simulink model "manual_steer"  (R2022b)
settings: Solver=ode4  StartTime=0.0  StopTime=100  RelTol=1e-3
model workspace (MAT data in the model file):
  x2xx = 0
undefined symbols (not defined in the file or in its folder): axle_rate_limit, BRAKE, brake_lag, brake_rate, DRIVE, KDspd, KIspd, KPspd, Lspd, Nspd, PARSa, PARSu, Q0, QD0, RW, Tb, Tmc, TOTALMASS, Tst, Uspd, v_ref
libraries: CarMaker4SL x72, slpidlib x4, TruckMaker4SL x1, simulink x1
(part 5 of 5)

== matlab function manual_steer/double sat_tyre general model/double-general-nonlineartyre-nonlinear-variable-matrix/M ==
  data: M output; q input
function M = calculate_M(q)

psi1 = q(3);
psi2 = q(4);
psi3 = q(5);

m1 = 11142;
m3 = 11142;
m2 = 7651; 
l_j1j2 = 11.4;
l_j2j3 = 9.4;
l_j1g1 = 5.862; 
l_j2g2 = 4.643; 
l_j3g3 = 5.538; 
iz1 = 143570; 
iz3 = 143570; 
iz2 = 37800;

l_kj = [l_j1g1, l_j1j2, l_j1j2;
             0, l_j2g2, l_j2j3;
             0,      0, l_j3g3;];
delta_kj = eye(3);
Jc = zeros(3, 5, 3);
for j = 1:3
    Jc(:, :, j) = [1, 0,  l_kj(1, j) * sin(psi1),  l_kj(2, j) * sin(psi2),  l_kj(3, j) * sin(psi3);
          0, 1, -l_kj(1, j) * cos(psi1), -l_kj(2, j) * cos(psi2), -l_kj(3, j) * cos(psi3);
          0, 0,          delta_kj(1, j),          delta_kj(2, j),          delta_kj(3, j);];
end

mj = [m1, m2, m3]';
izj = [iz1, iz2, iz3]';
Mj = zeros(3, 3, 3);
for j = 1:3
    Mj(:, :, j) = diag([mj(j), mj(j), izj(j)]);
end

M = zeros(5, 5);
for j = 1:3
    M = M + Jc(:, :, j)' * Mj(:, :, j) * Jc(:, :, j);
end

end

== matlab function manual_steer/double sat_tyre general model/double-general-nonlineartyre-nonlinear-variable-matrix/Tau_tire ==
  data: q input; qd input; delta input; Fx input; Tau_tire output; Alpha output
function [Tau_tire, Alpha] = calculate_Tau_tire(q, qd, delta, Fx)

% coefficient

l_j1j2 = 11.4;
l_j2j3 = 9.4;
l_j1a1 = 2.5;
l_j1a2 = 4;
l_j1a3 = 9.9;
l_j2a4 = 1.5;
l_j2a5 = 7.9;
l_j3a6 = 1.5;
l_j3a7 = 7.4;
l_j3a8 = 8.9;
h11 = 0.9625;
h12 = 0.9625;
h13 = 0.98;
h21 = 0.98; 
h22 = 0.98;
h31 = 0.98;
h32 = 0.9625;
h33 = 0.9625;

x = q(1);
y = q(2);
psi1 = q(3);
psi2 = q(4);
psi3 = q(5);
xd = qd(1);
yd = qd(2);
psi1d = qd(3);
psi2d = qd(4);
psi3d = qd(5);

psij = [psi1, psi2, psi3]';
Rot_w2v = zeros(2, 2, 3);
for i = 1:3
    Rot_w2v(:, :, i) = [cos(psij(i)), -sin(psij(i));
                        sin(psij(i)), cos(psij(i));];
end

Rot_v2t = zeros(2, 2, 8);
for i = 1:8
    Rot_v2t(:, :, i) = [cos(delta(i)), -sin(delta(i));
                        sin(delta(i)), cos(delta(i));];
end

xj = zeros(3, 1);
yj = zeros(3, 1);
xj(1) = x;
yj(1) = y;
xj(2) = x - l_j1j2*cos(psi1);
yj(2) = y - l_j1j2*sin(psi1);
xj(3) = x - l_j1j2*cos(psi1) - l_j2j3*cos(psi2);
yj(3) = y - l_j1j2*sin(psi1) - l_j2j3*sin(psi2);

u = zeros(2, 3);
n = zeros(2, 3);
for i = 1:3
    u(:, i)=[cos(q(i + 2)), sin(q(i + 2))]';
    n(:, i)=[-sin(q(i + 2)), cos(q(i + 2))]';
end

IU = [1, 1, 1, 2, 2, 3, 3, 3]';
l_ja = [l_j1a1, l_j1a2, l_j1a3, l_j2a4, l_j2a5, l_j3a6, l_j3a7, l_j3a8]';
ha = [h11, h12, h13, h21, h22, h31, h32, h33]';

L_long1 = [cos(psi1), cos(psi1), cos(psi1), cos(psi2), cos(psi2), cos(psi3), cos(psi3), cos(psi3);
           sin(psi1), sin(psi1), sin(psi1), sin(psi2), sin(psi2), sin(psi3), sin(psi3), sin(psi3);
           -h11, -h12, -h13, l_j1j2*sin(psi1-psi2), l_j1j2*sin(psi1-psi2), l_j1j2*sin(psi1-psi3), l_j1j2*sin(psi1-psi3), l_j1j2*sin(psi1-psi3);
           0, 0, 0, -h21, -h22, l_j2j3*sin(psi2-psi3), l_j2j3*sin(psi2-psi3), l_j2j3*sin(psi2-psi3);
           0, 0, 0, 0, 0, -h31, -h32, -h33;];

L_long2 = [cos(psi1), cos(psi1), cos(psi1), cos(psi2), cos(psi2), cos(psi3), cos(psi3), cos(psi3);
           sin(psi1), sin(psi1), sin(psi1), sin(psi2), sin(psi2), sin(psi3), sin(psi3), sin(psi3);
           h11, h12, h13, l_j1j2*sin(psi1-psi2), l_j1j2*sin(psi1-psi2), l_j1j2*sin(psi1-psi3), l_j1j2*sin(psi1-psi3), l_j1j2*sin(psi1-psi3);
           0, 0, 0, h21, h22, l_j2j3*sin(psi2-psi3), l_j2j3*sin(psi2-psi3), l_j2j3*sin(psi2-psi3);
           0, 0, 0, 0, 0, h31, h32, h33;];

L_lat1 = [-sin(psi1), -sin(psi1), -sin(psi1), -sin(psi2), -sin(psi2), -sin(psi3), -sin(psi3), -sin(psi3);
          cos(psi1), cos(psi1), cos(psi1), cos(psi2), cos(psi2), cos(psi3), cos(psi3), cos(psi3);
          -l_j1a1, -l_j1a2, -l_j1a3, -l_j1j2*cos(psi1-psi2), -l_j1j2*cos(psi1-psi2), -l_j1j2*cos(psi1-psi3), -l_j1j2*cos(psi1-psi3), -l_j1j2*cos(psi1-psi3);
          0, 0, 0, -l_j2a4, -l_j2a5, -l_j2j3*cos(psi2-psi3), -l_j2j3*cos(psi2-psi3), -l_j2j3*cos(psi2-psi3);
          0, 0, 0, 0, 0, -l_j3a6, -l_j3a7, -l_j3a8;];

L_lat2 = [-sin(psi1), -sin(psi1), -sin(psi1), -sin(psi2), -sin(psi2), -sin(psi3), -sin(psi3), -sin(psi3);
          cos(psi1), cos(psi1), cos(psi1), cos(psi2), cos(psi2), cos(psi3), cos(psi3), cos(psi3);
          -l_j1a1, -l_j1a2, -l_j1a3, -l_j1j2*cos(psi1-psi2), -l_j1j2*cos(psi1-psi2), -l_j1j2*cos(psi1-psi3), -l_j1j2*cos(psi1-psi3), -l_j1j2*cos(psi1-psi3);
          0, 0, 0, -l_j2a4, -l_j2a5, -l_j2j3*cos(psi2-psi3), -l_j2j3*cos(psi2-psi3), -l_j2j3*cos(psi2-psi3);
          0, 0, 0, 0, 0, -l_j3a6, -l_j3a7, -l_j3a8;];

Delta_c = zeros(8, 8);
Delta_s = zeros(8, 8);
for i = 1:8
    Delta_c(i, i) = cos(delta(i));
    Delta_s(i, i) = sin(delta(i));
end

vxj = zeros(3, 1);
vyj = zeros(3, 1);
vxj(1) = xd;
vyj(1) = yd;
vxj(2) = xd + l_j1j2*sin(psi1)*psi1d;
vyj(2) = yd - l_j1j2*cos(psi1)*psi1d;
vxj(3) = xd + l_j1j2*sin(psi1)*psi1d + l_j2j3*sin(psi2)*psi2d;
vyj(3) = yd - l_j1j2*cos(psi1)*psi1d - l_j2j3*cos(psi2)*psi2d;
va1 = zeros(2, 8);
va2 = zeros(2, 8);
psidj = [psi1d, psi2d, psi3d]';
for i = 1:8
    va1(:, i) = [vxj(IU(i)); vyj(IU(i))] - n(:, IU(i))*l_ja(i)*psidj(IU(i)) + (-1)*u(:, IU(i))*ha(i)*psidj(IU(i));
    va2(:, i) = [vxj(IU(i)); vyj(IU(i))] - n(:, IU(i))*l_ja(i)*psidj(IU(i)) + u(:, IU(i))*ha(i)*psidj(IU(i));
end

va1_v = zeros(2, 8);
va2_v = zeros(2, 8);
for i = 1:8
    va1_v(:, i) = inv(Rot_w2v(:, :, IU(i)))*va1(:, i);
    va2_v(:, i) = inv(Rot_w2v(:, :, IU(i)))*va2(:, i);
end

beta1 = zeros(8, 1);
beta2 = zeros(8, 1);
for i = 1:8
    beta1(i) = atan2(va1_v(2, i), va1_v(1, i));
    beta2(i) = atan2(va2_v(2, i), va2_v(1, i));
end

% magic formula
% 魔术公式参数
A = [1.65, -34, 1250, 4535, 12.8, 0.00501, -0.02103,  0.77394, ...
     0.0022890, 0.013442, 0.003709, 19.1656, 1.21356, 6.26206]';

% 轮胎垂向载荷 kN
Fz = 30000 / 1000;

Fy1 = zeros(8, 1);
Fy2 = zeros(8, 1);
gamma = 0;
for i = 1:8
    alpha = (delta(i) - beta1(i)) * 180 / pi;
    Sh = A(10) * Fz + A(11) + A(9) * gamma;
    Sv = A(12) * Fz * gamma + A(13) * Fz + A(14);
    C = A(1);
    D = A(2) * Fz ^ 2 + A(3) * Fz;
    BCD = A(4) * sin(2 * atan(Fz / A(5))) * (1 - A(6) * abs(gamma));
    B = BCD / (C * D);
    E = A(7) * Fz + A(8);
    x = alpha; % + Sh;
    % 轮胎侧向力
    Fy1(i) = D * sin(C * atan(B * x - E * (B * x - atan(B * x)))); % + Sv;
end
for i = 1:8
    alpha = (delta(i) - beta2(i)) * 180 / pi;
    Sh = A(10) * Fz + A(11) + A(9) * gamma;
    Sv = A(12) * Fz * gamma + A(13) * Fz + A(14);
    C = A(1);
    D = A(2) * Fz ^ 2 + A(3) * Fz;
    BCD = A(4) * sin(2 * atan(Fz / A(5))) * (1 - A(6) * abs(gamma));
    B = BCD / (C * D);
    E = A(7) * Fz + A(8);
    x = alpha; % + Sh;
    % 轮胎侧向力
    Fy2(i) = D * sin(C * atan(B * x - E * (B * x - atan(B * x)))); % + Sv;
end

Tau_tire = L_long1 * (Delta_c * Fx / 2 - Delta_s * Fy1) ...
         + L_long2 * (Delta_c * Fx / 2 - Delta_s * Fy2) ...
         + L_lat1 * (Delta_s * Fx / 2 + Delta_c * Fy1) ...
         + L_lat2 * (Delta_s * Fx / 2 + Delta_c * Fy2);

beta = (beta1 + beta2) / 2;
Alpha = delta - beta;

end

== matlab function manual_steer/double sat_tyre general model/double-general-nonlineartyre-nonlinear-variable-matrix/qdd ==
  data: M input; C input; D input; qd input; Q input; qdd output
function qdd = calculate_qdd(M, C, D, qd, Q)

qdd = inv(M)*(Q - C * qd - D * qd);

end

== matlab function manual_steer/single sat_tyre general model/single-general-lineartyre-variable/D ==
  data: D output
function D = calculate_D()

d1 = 10000;
d2 = 10000;

delta_kj = eye(3);
dj = [0, d1, d2, 0]';
D = zeros(5);

for k = 1:5
    for l = 1:5
        if k > 2 && l > 2
            if  l == k
                D(k, l) = (1 - delta_kj(1, k-2))*dj(k - 2) + (1 - delta_kj(3, k-2))*dj(k - 1);
            elseif l == k-1
                D(k, l) = -(1 - delta_kj(1, k-2))*dj(k - 2);
            elseif l == k+1
                D(k, l) = -(1 - delta_kj(3, k-2))*dj(k - 1);
            else
                D(k, l) = 0;
            end
        end
    end
end

end

== matlab function manual_steer/single sat_tyre general model/single-general-lineartyre-variable/M ==
  data: M output; q input
function M = calculate_M(q)

psi1 = q(3);
psi2 = q(4);
psi3 = q(5);

m1 = 11142;
m3 = 11142;
m2 = 7651; 
l_j1j2 = 11.4;
l_j2j3 = 9.4;
l_j1g1 = 5.862; 
l_j2g2 = 4.643; 
l_j3g3 = 5.538; 
iz1 = 143570; 
iz3 = 143570; 
iz2 = 37800;

l_kj = [l_j1g1, l_j1j2, l_j1j2;
             0, l_j2g2, l_j2j3;
             0,      0, l_j3g3;];
delta_kj = eye(3);
Jc = zeros(3, 5, 3);
for j = 1:3
    Jc(:, :, j) = [1, 0,  l_kj(1, j) * sin(psi1),  l_kj(2, j) * sin(psi2),  l_kj(3, j) * sin(psi3);
          0, 1, -l_kj(1, j) * cos(psi1), -l_kj(2, j) * cos(psi2), -l_kj(3, j) * cos(psi3);
          0, 0,          delta_kj(1, j),          delta_kj(2, j),          delta_kj(3, j);];
end

mj = [m1, m2, m3]';
izj = [iz1, iz2, iz3]';
Mj = zeros(3, 3, 3);
for j = 1:3
    Mj(:, :, j) = diag([mj(j), mj(j), izj(j)]);
end

M = zeros(5, 5);
for j = 1:3
    M = M + Jc(:, :, j)' * Mj(:, :, j) * Jc(:, :, j);
end

end

== matlab function manual_steer/double sat_tyre general model/ Motion Controller1/discrete-time subsystem/MATLAB Function ==
  data: str1 input; y output; PARSa input
function y = StrMux(str1,PARSa)
%distribute steering from driver (and auto steer in future versions)
y=PARSa(:,6);
y=y*str1;
end

== matlab function manual_steer/single sat_tyre general model/single-general-lineartyre-variable/Tau_tire ==
  data: q input; qd input; delta input; Fx input; Tau_tire output; Alpha output
function [Tau_tire, Alpha] = calculate_Tau_tire(q, qd, delta, Fx)

% coefficient

l_j1j2 = 11.4;
l_j2j3 = 9.4;
l_j1a1 = 2.5;
l_j1a2 = 4;
l_j1a3 = 9.9;
l_j2a4 = 1.5;
l_j2a5 = 7.9;
l_j3a6 = 1.5;
l_j3a7 = 7.4;
l_j3a8 = 8.9;
h11 = 0;
h12 = 0;
h13 = 0;
h21 = 0; 
h22 = 0;
h31 = 0;
h32 = 0;
h33 = 0;

ca_T = 3065;
ca1 = ca_T;
ca2 = ca_T;
ca3 = ca_T;
ca4 = ca_T;
ca5 = ca_T;
ca6 = ca_T;
ca7 = ca_T;
ca8 = ca_T;

psi1 = q(3);
psi2 = q(4);
psi3 = q(5);
xd = qd(1);
yd = qd(2);
psi1d = qd(3);
psi2d = qd(4);
psi3d = qd(5);

psij = [psi1, psi2, psi3]';
Rot_w2v = zeros(2, 2, 3);
for i = 1:3
    Rot_w2v(:, :, i) = [cos(psij(i)), -sin(psij(i));
                        sin(psij(i)), cos(psij(i));];
end

Rot_v2t = zeros(2, 2, 8);
for i = 1:8
    Rot_v2t(:, :, i) = [cos(delta(i)), -sin(delta(i));
                        sin(delta(i)), cos(delta(i));];
end

u = zeros(2, 3);
n = zeros(2, 3);
for i = 1:3
    u(:, i)=[cos(q(i + 2)), sin(q(i + 2))]';
    n(:, i)=[-sin(q(i + 2)), cos(q(i + 2))]';
end

IU = [1, 1, 1, 2, 2, 3, 3, 3]';
l_ja = [l_j1a1, l_j1a2, l_j1a3, l_j2a4, l_j2a5, l_j3a6, l_j3a7, l_j3a8]';
ha = [h11, h12, h13, h21, h22, h31, h32, h33]';

L_long1 = [cos(psi1), cos(psi1), cos(psi1), cos(psi2), cos(psi2), cos(psi3), cos(psi3), cos(psi3);
           sin(psi1), sin(psi1), sin(psi1), sin(psi2), sin(psi2), sin(psi3), sin(psi3), sin(psi3);
           -h11, -h12, -h13, l_j1j2*sin(psi1-psi2), l_j1j2*sin(psi1-psi2), l_j1j2*sin(psi1-psi3), l_j1j2*sin(psi1-psi3), l_j1j2*sin(psi1-psi3);
           0, 0, 0, -h21, -h22, l_j2j3*sin(psi2-psi3), l_j2j3*sin(psi2-psi3), l_j2j3*sin(psi2-psi3);
           0, 0, 0, 0, 0, -h31, -h32, -h33;];

L_long2 = [cos(psi1), cos(psi1), cos(psi1), cos(psi2), cos(psi2), cos(psi3), cos(psi3), cos(psi3);
           sin(psi1), sin(psi1), sin(psi1), sin(psi2), sin(psi2), sin(psi3), sin(psi3), sin(psi3);
           h11, h12, h13, l_j1j2*sin(psi1-psi2), l_j1j2*sin(psi1-psi2), l_j1j2*sin(psi1-psi3), l_j1j2*sin(psi1-psi3), l_j1j2*sin(psi1-psi3);
           0, 0, 0, h21, h22, l_j2j3*sin(psi2-psi3), l_j2j3*sin(psi2-psi3), l_j2j3*sin(psi2-psi3);
           0, 0, 0, 0, 0, h31, h32, h33;];

L_lat1 = [-sin(psi1), -sin(psi1), -sin(psi1), -sin(psi2), -sin(psi2), -sin(psi3), -sin(psi3), -sin(psi3);
          cos(psi1), cos(psi1), cos(psi1), cos(psi2), cos(psi2), cos(psi3), cos(psi3), cos(psi3);
          -l_j1a1, -l_j1a2, -l_j1a3, -l_j1j2*cos(psi1-psi2), -l_j1j2*cos(psi1-psi2), -l_j1j2*cos(psi1-psi3), -l_j1j2*cos(psi1-psi3), -l_j1j2*cos(psi1-psi3);
          0, 0, 0, -l_j2a4, -l_j2a5, -l_j2j3*cos(psi2-psi3), -l_j2j3*cos(psi2-psi3), -l_j2j3*cos(psi2-psi3);
          0, 0, 0, 0, 0, -l_j3a6, -l_j3a7, -l_j3a8;];

L_lat2 = [-sin(psi1), -sin(psi1), -sin(psi1), -sin(psi2), -sin(psi2), -sin(psi3), -sin(psi3), -sin(psi3);
          cos(psi1), cos(psi1), cos(psi1), cos(psi2), cos(psi2), cos(psi3), cos(psi3), cos(psi3);
          -l_j1a1, -l_j1a2, -l_j1a3, -l_j1j2*cos(psi1-psi2), -l_j1j2*cos(psi1-psi2), -l_j1j2*cos(psi1-psi3), -l_j1j2*cos(psi1-psi3), -l_j1j2*cos(psi1-psi3);
          0, 0, 0, -l_j2a4, -l_j2a5, -l_j2j3*cos(psi2-psi3), -l_j2j3*cos(psi2-psi3), -l_j2j3*cos(psi2-psi3);
          0, 0, 0, 0, 0, -l_j3a6, -l_j3a7, -l_j3a8;];

Delta_c = zeros(8, 8);
Delta_s = zeros(8, 8);
for i = 1:8
    Delta_c(i, i) = cos(delta(i));
    Delta_s(i, i) = sin(delta(i));
end

vxj = zeros(3, 1);
vyj = zeros(3, 1);
vxj(1) = xd;
vyj(1) = yd;
vxj(2) = xd + l_j1j2*sin(psi1)*psi1d;
vyj(2) = yd - l_j1j2*cos(psi1)*psi1d;
vxj(3) = xd + l_j1j2*sin(psi1)*psi1d + l_j2j3*sin(psi2)*psi2d;
vyj(3) = yd - l_j1j2*cos(psi1)*psi1d - l_j2j3*cos(psi2)*psi2d;
va1 = zeros(2, 8);
va2 = zeros(2, 8);
psidj = [psi1d, psi2d, psi3d]';
for i = 1:8
    va1(:, i) = [vxj(IU(i)); vyj(IU(i))] - n(:, IU(i))*l_ja(i)*psidj(IU(i)) + (-1)*u(:, IU(i))*ha(i)*psidj(IU(i));
    va2(:, i) = [vxj(IU(i)); vyj(IU(i))] - n(:, IU(i))*l_ja(i)*psidj(IU(i)) + u(:, IU(i))*ha(i)*psidj(IU(i));
end

va1_v = zeros(2, 8);
va2_v = zeros(2, 8);
for i = 1:8
    va1_v(:, i) = inv(Rot_w2v(:, :, IU(i)))*va1(:, i);
    va2_v(:, i) = inv(Rot_w2v(:, :, IU(i)))*va2(:, i);
end

beta1 = zeros(8, 1);
beta2 = zeros(8, 1);
for i = 1:8
    beta1(i) = atan2(va1_v(2, i), va1_v(1, i));
    beta2(i) = atan2(va2_v(2, i), va2_v(1, i));
end

ca = [ca1, ca2, ca3, ca4, ca5, ca6, ca7, ca8]';
Ca = diag(ca);

sat = 10;
alpha1 = delta - beta1;
alpha2 = delta - beta2;
for i = 1:8
    if abs(alpha1(i)) > sat * pi / 180
        alpha1(i) = sign(alpha1(i)) * sat * pi / 180;
    end
    if abs(alpha2(i)) > sat * pi / 180
        alpha2(i) = sign(alpha2(i)) * sat * pi / 180;
    end
end

Tau_tire = L_long1 * (Delta_c * Fx / 2 - Delta_s * Ca * alpha1) ...
         + L_long2 * (Delta_c * Fx / 2 - Delta_s * Ca * alpha2) ...
         + L_lat1 * (Delta_s * Fx / 2 + Delta_c * Ca * alpha1) ...
         + L_lat2 * (Delta_s * Fx / 2 + Delta_c * Ca * alpha2);

beta = (beta1 + beta2) / 2;
Alpha = delta - beta;

end

== matlab function manual_steer/double sat_tyre general model/ Motion Controller/discrete-time subsystem/getU ==
  settings: updateMethod=DISCRETE
  data: U output; q input; qd input
function U = vx_conversion(q, qd)

% convert q and qd to vx6 needed for the driver model

% nominal point P of driver
xxp = 2;  
u1 = [cos(q(3)); sin(q(3))];
n1 = [-sin(q(3)); cos(q(3))];

% global velocity at front joint
vj1 = qd(1:2); 

% move to driver point
vp = vj1 - qd(3)*xxp*n1; 

% components in body axes (unit 1)
U = dot(vp, u1);

end

== matlab function manual_steer/double sat_tyre general model/double-general-lineartyre-variable/状态输入 ==
  data: steer input; sign output; fx input
function sign = is_start(steer, fx)

sign = 1;
if steer == zeros(8,1) 
    if fx == zeros(8,1)
        sign = 0;
    end
end

end

== matlab function manual_steer/single sat_tyre general model/single-general-lineartyre-variable/qdd ==
  data: M input; C input; D input; qd input; Q input; qdd output
function qdd = calculate_qdd(M, C, D, qd, Q)

qdd = inv(M)*(Q - C * qd - D * qd);

end

== matlab function manual_steer/single sat_tyre general model/single-general-lineartyre-variable/状态输入 ==
  data: steer input; sign output; fx input
function sign = is_start(steer, fx)

sign = 1;
if steer == zeros(8,1) 
    if fx == zeros(8,1)
        sign = 0;
    end
end

end

== matlab function manual_steer/newton sat_tyre linear model/newton sat_tyre linear/get tyre f ==
  data: q_input input; yij output; qd_input input; delta_input input
function yij = get_tyre_f(q_input, qd_input, delta_input)

% the number of vehicle units
unit_n = 3;
% the number of vehicle axles
axle_m = 8;
% the unit of the respective axle
getNumUnit = [1, 1, 1, 2, 2, 3, 3, 3];


% the tire cornering stiffness
Ca = 3065; % * 180 / pi;

% the length of every vehicle unit
lu = [11.4, 9.4, 11.4];
% the length of every vehicle unit from the front joint to the mass center
lg = [5.862, 4.643, 5.538];
% the length of every vehicle unit from the front joint to the axle center
la = [2.5, 4, 9.9, 1.5, 7.9, 1.5, 7.4, 8.9];

sat = 10;

% calculate U \beta r \theta
psi = q_input(3:unit_n+2);
dpsi = qd_input(3:unit_n+2);
delta = delta_input;

theta = zeros(unit_n-1, 1);
for i = 1:unit_n-1
    theta(i) = psi(i) - psi(i+1);
end

v_gw = zeros(2, unit_n);
v_gv = zeros(2, unit_n);
v_jw = zeros(2, unit_n);
beta = zeros(unit_n, 1);

v_jw(:, 1) = qd_input(1:2);
for i = 1:unit_n-1
    v_jw(1, i+1) = v_jw(1, i) + sin(psi(i)) * lu(i) * dpsi(i);
    v_jw(2, i+1) = v_jw(2, i) - cos(psi(i)) * lu(i) * dpsi(i);
end

for i = 1:unit_n
    v_gw(1, i) = v_jw(1, i) + sin(psi(i)) * lg(i) * dpsi(i);
    v_gw(2, i) = v_jw(2, i) - cos(psi(i)) * lg(i) * dpsi(i);
    v_gv(1, i) = v_gw(1, i) * cos(psi(i)) + v_gw(2, i) * sin(psi(i));
    v_gv(2, i) = -v_gw(1, i) * sin(psi(i)) + v_gw(2, i) * cos(psi(i));
    U = v_gv(1, 1);
    beta(i) = v_gv(2, i) / U;
end

% judge the slip angle 

v_aw = zeros(2, axle_m);
v_av = zeros(2, axle_m);
beta_a = zeros(axle_m, 1);
for i = 1:axle_m
    v_aw(1, i) = v_jw(1, getNumUnit(i)) + sin(psi(getNumUnit(i))) * la(getNumUnit(i)) * dpsi(getNumUnit(i));
    v_aw(2, i) = v_jw(2, getNumUnit(i)) - cos(psi(getNumUnit(i))) * la(getNumUnit(i)) * dpsi(getNumUnit(i));
    v_av(1, i) = v_aw(1, i) * cos(psi(getNumUnit(i))) + v_aw(2, i) * sin(psi(getNumUnit(i)));
    v_av(2, i) = -v_aw(1, i) * sin(psi(getNumUnit(i))) + v_aw(2, i) * cos(psi(getNumUnit(i)));
    beta_a(i) = v_av(2, i) / U;
end

alpha = delta - beta_a;
for i = 1:8
    if abs(alpha(i)) > sat * pi / 180
        alpha(i) = sign(alpha(i)) * sat * pi / 180;
    end
end

yij = Ca * alpha;

end

== matlab function manual_steer/newton sat_tyre linear model/proc/MatMaker ==
  data: Va output; Vaa output; Vj output; q input; qd input; Vg output; PARSu input; PARSa input; Vgg output
function [Va,Vaa,Vj,Vg,Vgg] =Vmaker(q,qd,PARSu,PARSa)


%%%%%%%%%%%%%%%%%%%%%%%%%%%%%%%%%%%%%%%%%%%%%%%%%%%%%%%%%%%%%%%%%%%%%%%%%

Va=zeros(2,8); % (2,Na) - axle velocities in globals
Vj=zeros(2,4); % (2,Nu+1) - joint velocities in globals
Vg=zeros(2,3); % (2,Nu) - CG velocities in globals
%%%%%%%%%%%%%%%%%%%%%%%%%%%%%%%%%%%%%%%%%%%%%%%%%%%%%%%%%%%%%%%%%%%%%%%%%%
Vaa=Va; % axle velocities in locals
Vgg=Vg; % CG velocities in locals

% actual dimensions
Nu=size(PARSu,1);
Na=size(PARSa,1);

LL=PARSu(:,3);
XG=PARSu(:,4);
XX=LL-XG;

uu=zeros(2,Nu); 
nn=zeros(2,Nu);
for i=1:Nu
    c=cos(q(i+2));s=sin(q(i+2));
    uu(:,i)=[c,s]';
    nn(:,i)=[-s,c]';
end


Vj(:,1)=[qd(1),qd(2)]';
for i=1:Nu
    Vj(:,i+1)=Vj(:,i)-qd(i+2)*LL(i)*nn(:,i);%negative sign since working backwards
    Vg(:,i)=Vj(:,i)-qd(i+2)*XX(i)*nn(:,i);
    Vgx=dot(Vg(:,i),uu(:,i));Vgy=dot(Vg(:,i),nn(:,i));
    Vgg(:,i)=[Vgx;Vgy];
end

%velocities at axles 
for i=1:Na
    xa=PARSa(i,1);
    k=PARSa(i,2);
    Va(:,i)=Vj(:,k+1)+qd(k+2)*xa*nn(:,k);
    Vax=dot(Va(:,i),uu(:,k));Vay=dot(Va(:,i),nn(:,k));
    Vaa(:,i)=[Vax;Vay];
end

== matlab function manual_steer/newton sat_tyre linear model/newton sat_tyre linear/state_update ==
  data: x input; q_input input; qdd_output output; qd_input input; yij input
function qdd_output = get_state(x, q_input, qd_input, yij)

% the number of vehicle units
unit_n = 3;
% the number of vehicle axles
axle_m = 8;
% the unit of the respective axle
getNumUnit = [1, 1, 1, 2, 2, 3, 3, 3];

% the mass of every vehicle unit
m = [11142, 7651, 11142];
% the rotational inertia of every vehicle unit
Iz = [143570, 37800, 143570];
% the tire cornering stiffness
Ca = 3065; % * 180 / pi;

% the length of every vehicle unit
lu = [11.4, 9.4, 11.4];
% the length of every vehicle unit from the front joint to the mass center
lg = [5.862, 4.643, 5.538];
% the length of every vehicle unit from the front joint to the axle center
la = [2.5, 4, 9.9, 1.5, 7.9, 1.5, 7.4, 8.9];

% calculate U \beta r \theta
psi = q_input(3:unit_n+2);
dpsi = qd_input(3:unit_n+2);

v_gw = zeros(2, unit_n);
v_gv = zeros(2, unit_n);
v_jw = zeros(2, unit_n);
beta = zeros(unit_n, 1);

v_jw(:, 1) = qd_input(1:2);
for i = 1:unit_n-1
    v_jw(1, i+1) = v_jw(1, i) + sin(psi(i)) * lu(i) * dpsi(i);
    v_jw(2, i+1) = v_jw(2, i) - cos(psi(i)) * lu(i) * dpsi(i);
end

for i = 1:unit_n
    v_gw(1, i) = v_jw(1, i) + sin(psi(i)) * lg(i) * dpsi(i);
    v_gw(2, i) = v_jw(2, i) - cos(psi(i)) * lg(i) * dpsi(i);
    v_gv(1, i) = v_gw(1, i) * cos(psi(i)) + v_gw(2, i) * sin(psi(i));
    v_gv(2, i) = -v_gw(1, i) * sin(psi(i)) + v_gw(2, i) * cos(psi(i));
    U = v_gv(1, 1);
    beta(i) = v_gv(2, i) / U;
end

% newton 
L = cell(1, unit_n);
for k = 1:unit_n
    % L1: 各轴中心到单元质心的距离，前为正，后为负
    L1 = lg(k) - la(getNumUnit == k);
    L{k} = L1;
end

nx = 3*unit_n-1; % number of states
nv = 4*unit_n-2; % number of variables (including joint forces)

% S * (\dot{x} R)' + P x = By y 方程
% x = {\beta r \theta}  n n n-1 状态量
% r = \dot{\psi} 横摆角速度
% \theta = \psi_j - \psi_j+1  铰接角

% dimensions of primary matrices
S = zeros(nv, nv);
P = zeros(nv, nx);
BY = zeros(nv, axle_m);
K1 = zeros(axle_m, nx);
K2 = zeros(axle_m, axle_m);

% joint damp
% input matrix for external yaw moments
BM = zeros(nv, unit_n); 

% populate S,P,B equation-by-equation

% first define end-index of sub-matrix blocks
% 3n-1个状态，前n个是质心侧偏角，中间n个是横摆角速度，最后n-1个是铰接角
b1 = unit_n;         % last row of beta_dot
b2 = 2 * unit_n;     % last row of r_dot
b3 = 3 * unit_n - 1; % last row of theta_dot

% also need number of 'preceding' axles at each unit
% 每个单元前面所有的单元共有多少个轴
pax = zeros(1, unit_n); % preceding axle numbers
for i = 2:unit_n
    pax(i) = pax(i - 1) + length(L{i - 1});
end

% equation (1)
for i = 1:unit_n 
    S(i, i) = m(i) * U;
    P(i, b1 + i) = m(i) * U;
    if i > 1
        % R_(i - 1) term in equ(1)
        S(i, b3 + i - 1) = -1;
    end 
    if i < unit_n
        % R_i term 
        S(i, b3 + i) = 1;
    end 
    for j = 1:length(L{i})
        % Yij terms
       BY(i, pax(i) + j) = 1; 
    end
end

% equation (2)
for i = 1:unit_n 
    S(b1 + i, b1 + i) = Iz(i);
    if i > 1
        % R_(i-1) term in equ(1)
        S(b1 + i, b3 + i - 1) = -lg(i);
    end 
    if i < unit_n
        % R_i term 
        S(b1 + i, b3 + i) = lg(i) - lu(i);
    end 
    for j = 1:length(L{i})
        % Mij terms
       BY(b1 + i, pax(i) + j) = L{i}(j); 
    end
    BM(b1+i) = 1; % direct yaw moment term
end

% equation (3)
for i = 1:unit_n-1
    % theta-dot term
    S(b2 + i, b2 + i) = 1; 
    % r_i in notes = unit in front of the joint
    P(b2 + i, b1 + i) = -1; 
    % r_(i+1)
    P(b2 + i, b1 + i + 1) = 1; 
end

% equation (4) 
for i = 1:unit_n-1 
    S(b3 + i, i + 1) = U;
    S(b3 + i, i) = -U; 
    S(b3 + i, b1 + i + 1) = lg(i + 1);
    S(b3 + i, b1 + i) = -(lg(i) - lu(i));
    S(b3 + i, b2 + i) = -U; 
end

% K1 matrix, Y = K1 * X for each axle force
for i = 1:unit_n
    for j = 1:length(L{i})
        % 'flat' axle index
        ia = pax(i) + j; 
        K1(ia, i) = U;
        K1(ia, b1 + i) = L{i}(j);
        K1(ia, :) = -K1(ia, :) * Ca / U;
    end
end

% K2 matrix, go axle by axle
for i = 1:unit_n
    for j = 1:length(L{i})
        % 'flat' axle index
        ia = pax(i) + j; 
        K2(ia, ia) = Ca;
    end
end

dxx = S \ (BY * yij - P * x);
dx= dxx(1:nx, :);

% dx to new qdd
dbeta_1 = dx(1);
qdd_v = zeros(2, 1);
qdd_v(1) = 0;
qdd_v(2) = dbeta_1 * U + lg(1) * dx(unit_n+1) + dx(unit_n+1) * U;

qd_v = zeros(2, 1);
qd_v(1) = qd_input(1) * cos(psi(1)) + qd_input(2) * sin(psi(1));
qd_v(2) = -qd_input(1) * sin(psi(1)) + qd_input(2) * cos(psi(1));
Twv = [cos(psi(1)), -sin(psi(1));
     sin(psi(1)), cos(psi(1))];
Tdwv = [-sin(psi(1))*dpsi(1), -cos(psi(1))*dpsi(1);
        cos(psi(1))*dpsi(1), -sin(psi(1))*dpsi(1)];

qdd_output = zeros(unit_n+2, 1);
qdd_output(1:2) = Twv * qdd_v + Tdwv * qd_v;
qdd_output(3:unit_n+2) = dx(unit_n+1:2*unit_n);

end

== matlab function manual_steer/kinetic model/ Motion Controller No Fx/MATLAB Function ==
  data: str1 input; y output; PARSa input
function y = StrMux(str1,PARSa)

% distribute steering from driver (and auto steer in future versions)
y = PARSa(:,6);
y = y*str1;

end

== matlab function manual_steer/kinetic model/kinetic linear/状态更新 ==
  data: q input; v_ref input; delta input; qd_output output; qd input
function qd_output = kinetic_model(q, v_ref, delta, qd)

psi1 = q(3);
psi2 = q(4);
psi3 = q(5);

% fixed parameter
l_g1j2 = 5.538;
l_j2g2 = 9.4 - 4.757;
l_g2j3 = 4.757;
l_a1a3 = 7.4;
l_a4a5 = 6.4;
l_a6a8 = 7.4;

% 假设所有车体都有侧偏，即速度方向与运动方向不同
% 输入为vx1, vy1, x, y, psi1, psi2, psi3, delta
vx1 = v_ref;
vy1 = 0;
% vx1 = vxg * cos(psi1) + vyg * sin(psi1);
% vy1 = -vxg * sin(psi1) + vyg * cos(psi1);

vx = vx1 * cos(psi1) - vy1 * sin(psi1);
vy = vx1 * sin(psi1) + vy1 * cos(psi1);

% disp(delta);

% 目标为xd, yd, psi1d, psi2d, psi3d
psi1d = vx1 * (tan(delta(1)) + tan(delta(3))) / l_a1a3;
vx2 = vx1 * cos(psi1 - psi2) + (-vy1 + l_g1j2 * psi1d) * sin(psi1 - psi2);
psi2d = vx2 * (tan(delta(4)) + tan(delta(5))) / l_a4a5;
vy2 = vx1 * sin(psi1 - psi2) - (-vy1 + l_g1j2 * psi1d) * cos(psi1 - psi2) - l_j2g2 * psi2d;
vx3 = vx2 * cos(psi2 - psi3) + (-vy2 + l_g2j3 * psi2d) * sin(psi2 - psi3);
psi3d = vx3 * (tan(delta(6)) + tan(delta(8))) / l_a6a8;

xd = vx - 5.862 * sin(psi1) * psi1d;
yd = vy + 5.862 * cos(psi1) * psi1d;
% xd = qd(1);
% yd = qd(2);

qd_output = [xd; yd; psi1d; psi2d; psi3d];

% qd_output = zeros(5, 1);

== matlab function manual_steer/double sat_tyre general model/double-general-lineartyre-variable/C ==
  data: q input; qd input; C output
function C = calculate_C(q, qd)

m1 = 11142;
m3 = 11142;
m2 = 7651; 
l_j1j2 = 11.4;
l_j2j3 = 9.4;
l_j1g1 = 5.862; 
l_j2g2 = 4.643; 
l_j3g3 = 5.538; 

psi1 = q(3);
psi2 = q(4);
psi3 = q(5);
xd = qd(1);
yd = qd(2);
psi1d = qd(3);
psi2d = qd(4);
psi3d = qd(5);

C = [0, 0, (l_j1g1*m1 + l_j1j2*(m2 + m3))*cos(psi1)*psi1d, (l_j2g2*m2 + l_j2j3*m3)*cos(psi2)*psi2d, l_j3g3*m3*cos(psi3)*psi3d;
     0, 0, (l_j1g1*m1 + l_j1j2*(m2 + m3))*sin(psi1)*psi1d, (l_j2g2*m2 + l_j2j3*m3)*sin(psi2)*psi2d, l_j3g3*m3*sin(psi3)*psi3d;
     1/2*(l_j1g1*m1 + l_j1j2*(m2 + m3))*cos(psi1)*psi1d, 1/2*(l_j1g1*m1 + l_j1j2*(m2 + m3))*sin(psi1)*psi1d, -1/2*(l_j1g1*m1 + l_j1j2*(m2 + m3))*(xd*cos(psi1)+yd*sin(psi1))+1/2*(l_j2g2*l_j1j2*m2+l_j1j2*l_j2j3*m3)*sin(psi1-psi2)*psi2d+1/2*l_j3g3*l_j1j2*m3*sin(psi1-psi3)*psi3d, (l_j2g2*l_j1j2*m2+l_j1j2*l_j2j3*m3)*sin(psi1-psi2)*(-1/2*psi1d+psi2d), l_j3g3*l_j1j2*m3*sin(psi1-psi3)*(-1/2*psi1d+psi3d);
     1/2*(l_j2g2*m2 + l_j2j3*m3)*cos(psi2)*psi2d, 1/2*(l_j2g2*m2 + l_j2j3*m3)*sin(psi2)*psi2d, (l_j2g2*l_j1j2*m2+l_j1j2*l_j2j3*m3)*sin(psi1-psi2)*(-psi1d+1/2*psi2d), -1/2*(l_j2g2*m2+l_j2j3*m3)*(xd*cos(psi2)+yd*sin(psi2))-1/2*(l_j2g2*l_j1j2*m2+l_j1j2*l_j2j3*m3)*sin(psi1-psi2)*psi1d+1/2*l_j3g3*l_j2j3*m3*sin(psi2-psi3)*psi3d, l_j3g3*l_j2j3*m3*sin(psi2-psi3)*(-1/2*psi2d+psi3d);
     1/2*l_j3g3*m3*cos(psi3)*psi3d, 1/2*l_j3g3*m3*sin(psi3)*psi3d, l_j3g3*l_j1j2*m3*sin(psi1-psi3)*(-psi1d+1/2*psi3d), l_j3g3*l_j2j3*m3*sin(psi2-psi3)*(-psi2d+1/2*psi3d), -1/2*l_j3g3*m3*(xd*cos(psi3)+yd*sin(psi3))-1/2*l_j3g3*l_j1j2*m3*sin(psi1-psi3)*psi1d-1/2*l_j3g3*l_j2j3*m3*sin(psi2-psi3)*psi2d;];

end

== matlab function manual_steer/kinetic model/kinetic linear/状态输入 ==
  data: steer input; sign output
function sign = is_start(steer)

sign = 1;
if steer == zeros(8,1) 
    sign = 0;
end

end

== matlab function manual_steer/truckmaker model/TruckMaker/IPG Vehicle/AFGc/MATLAB Function ==
  data: str1 input; y output; PARSa input
function y = StrMux(str1,PARSa)
%distribute steering from driver (and auto steer in future versions)
y=PARSa(:,6);
y=y*str1;
end

== matlab function manual_steer/newton sat_tyre linear model/newton sat_tyre linear/状态输入 ==
  data: steer input; sign output
function sign = is_start(steer)

sign = 1;
if steer == zeros(8,1) 
    sign = 0;
end

end

== matlab function manual_steer/truckmaker model/TruckMaker/IPG Vehicle/AFGc/find_vx ==
  settings: updateMethod=DISCRETE
  data: vx6 output; q input; qd input
function vx6 = vx_conversion(q,qd)
%#codegen
% convert q and qd to vx6 needed for the driver model

xxp=2; %nominal point P of driver 
u1=[cos(q(3));sin(q(3))];n1=[-sin(q(3));cos(q(3))];
rp = q(1:2)-xxp*u1;

v00=qd(1:2); %global velocity at front joint
vp=v00-qd(3)*xxp*n1; %move to driver point
U=dot(vp,u1);V=dot(vp,n1); %components in body axes (unit 1)
vx6=[U;V;qd(3);rp;q(3)]; %standard format ... [U,V,r,x,y,psi]'
end

== matlab function manual_steer/kinetic model/proc/MatMaker ==
  data: Va output; Vaa output; Vj output; q input; qd input; Vg output; PARSu input; PARSa input; Vgg output
function [Va,Vaa,Vj,Vg,Vgg] =Vmaker(q,qd,PARSu,PARSa)


%%%%%%%%%%%%%%%%%%%%%%%%%%%%%%%%%%%%%%%%%%%%%%%%%%%%%%%%%%%%%%%%%%%%%%%%%

Va=zeros(2,8); % (2,Na) - axle velocities in globals
Vj=zeros(2,4); % (2,Nu+1) - joint velocities in globals
Vg=zeros(2,3); % (2,Nu) - CG velocities in globals
%%%%%%%%%%%%%%%%%%%%%%%%%%%%%%%%%%%%%%%%%%%%%%%%%%%%%%%%%%%%%%%%%%%%%%%%%%
Vaa=Va; % axle velocities in locals
Vgg=Vg; % CG velocities in locals

% actual dimensions
Nu=size(PARSu,1);
Na=size(PARSa,1);

LL=PARSu(:,3);
XG=PARSu(:,4);
XX=LL-XG;

uu=zeros(2,Nu); 
nn=zeros(2,Nu);
for i=1:Nu
    c=cos(q(i+2));s=sin(q(i+2));
    uu(:,i)=[c,s]';
    nn(:,i)=[-s,c]';
end


Vj(:,1)=[qd(1),qd(2)]';
for i=1:Nu
    Vj(:,i+1)=Vj(:,i)-qd(i+2)*LL(i)*nn(:,i);%negative sign since working backwards
    Vg(:,i)=Vj(:,i)-qd(i+2)*XX(i)*nn(:,i);
    Vgx=dot(Vg(:,i),uu(:,i));Vgy=dot(Vg(:,i),nn(:,i));
    Vgg(:,i)=[Vgx;Vgy];
end

%velocities at axles 
for i=1:Na
    xa=PARSa(i,1);
    k=PARSa(i,2);
    Va(:,i)=Vj(:,k+1)+qd(k+2)*xa*nn(:,k);
    Vax=dot(Va(:,i),uu(:,k));Vay=dot(Va(:,i),nn(:,k));
    Vaa(:,i)=[Vax;Vay];
end

== matlab function manual_steer/truckmaker model/TruckMaker/IPG Vehicle/AFGc/proc/MatMaker ==
  data: Va output; Vaa output; Vj output; q input; qd input; Vg output; PARSu input; PARSa input; Vgg output
function [Va,Vaa,Vj,Vg,Vgg] =Vmaker(q,qd,PARSu,PARSa)


%%%%%%%%%%%%%%%%%%%%%%%%%%%%%%%%%%%%%%%%%%%%%%%%%%%%%%%%%%%%%%%%%%%%%%%%%

Va=zeros(2,8); % (2,Na) - axle velocities in globals
Vj=zeros(2,4); % (2,Nu+1) - joint velocities in globals
Vg=zeros(2,3); % (2,Nu) - CG velocities in globals
%%%%%%%%%%%%%%%%%%%%%%%%%%%%%%%%%%%%%%%%%%%%%%%%%%%%%%%%%%%%%%%%%%%%%%%%%%
Vaa=Va; % axle velocities in locals
Vgg=Vg; % CG velocities in locals

% actual dimensions
Nu=size(PARSu,1);
Na=size(PARSa,1);

LL=PARSu(:,3);
XG=PARSu(:,4);
XX=LL-XG;

uu=zeros(2,Nu); 
nn=zeros(2,Nu);
for i=1:Nu
    c=cos(q(i+2));s=sin(q(i+2));
    uu(:,i)=[c,s]';
    nn(:,i)=[-s,c]';
end


Vj(:,1)=[qd(1),qd(2)]';
for i=1:Nu
    Vj(:,i+1)=Vj(:,i)-qd(i+2)*LL(i)*nn(:,i);%negative sign since working backwards
    Vg(:,i)=Vj(:,i)-qd(i+2)*XX(i)*nn(:,i);
    Vgx=dot(Vg(:,i),uu(:,i));Vgy=dot(Vg(:,i),nn(:,i));
    Vgg(:,i)=[Vgx;Vgy];
end

%velocities at axles 
for i=1:Na
    xa=PARSa(i,1);
    k=PARSa(i,2);
    Va(:,i)=Vj(:,k+1)+qd(k+2)*xa*nn(:,k);
    Vax=dot(Va(:,i),uu(:,k));Vay=dot(Va(:,i),nn(:,k));
    Vaa(:,i)=[Vax;Vay];
end

== matlab function manual_steer/truckmaker model/TruckMaker/IPG Vehicle/AFGc/q&qd builder/build q/generate q ==
  data: FR1x input; q output; FR1y input; u1_yaw input; u2_yaw input; u3_yaw input
function q =generate_q(FR1x,FR1y,u1_yaw,u2_yaw,u3_yaw)

l=11.4;%FR1 of u1 to front reference point


q=zeros(5,1);
q(1)=FR1x+l*cos(u1_yaw);
q(2)=FR1y+l*sin(u1_yaw);
q(3)=u1_yaw;
q(4)=u2_yaw;
q(5)=u3_yaw;
end

== matlab function manual_steer/truckmaker model/TruckMaker/IPG Vehicle/AFGc/q&qd builder/build qd/generate qd ==
  data: vxFR1 input; q_d output; vyFR1 input; u1_yaw_rate input; u2_yaw_rate input; u3_yaw_rate input; u1_yaw_angle input
function q_d =generate_qd(vxFR1,vyFR1,u1_yaw_rate,u2_yaw_rate,u3_yaw_rate, u1_yaw_angle)

l=11.4;%FR1 of u1 to front reference point

q_d=zeros(5,1);

u1=[cos(u1_yaw_angle);sin(u1_yaw_angle)];n1=[-sin(u1_yaw_angle);cos(u1_yaw_angle)];

vfr1=[vxFR1;vyFR1];
q_d(1:2)=vfr1+u1_yaw_rate*l*n1;
% q_d(1)=vxFR1-l*u1_yaw_rate*cos(u1_yaw_angle);
% q_d(2)=vyFR1+l*u1_yaw_rate*sin(u1_yaw_angle);
q_d(3)=u1_yaw_rate;
q_d(4)=u2_yaw_rate;
q_d(5)=u3_yaw_rate;

end

== matlab function manual_steer/single sat_tyre general model/ Motion Controller/discrete-time subsystem single/MATLAB Function1 ==
  data: adem input; y output; PARSu input; PARSa input
function y = wheel_force_distibution(adem,PARSu,PARSa)

y=zeros(8,1); 
mass=sum(PARSu(:,1));
Na=size(PARSa,1);
if adem>0
    y(1:Na)=PARSa(:,4); %drive axle distribution
else
    y(1:Na)=PARSa(:,5); %brake force distribution
end
n=sum(y);
y=y*mass*adem/n;
end

== matlab function manual_steer/single sat_tyre general model/proc/MatMaker ==
  data: Va output; Vaa output; Vj output; q input; qd input; Vg output; PARSu input; PARSa input; Vgg output
function [Va,Vaa,Vj,Vg,Vgg] =Vmaker(q,qd,PARSu,PARSa)


%%%%%%%%%%%%%%%%%%%%%%%%%%%%%%%%%%%%%%%%%%%%%%%%%%%%%%%%%%%%%%%%%%%%%%%%%

Va=zeros(2,8); % (2,Na) - axle velocities in globals
Vj=zeros(2,4); % (2,Nu+1) - joint velocities in globals
Vg=zeros(2,3); % (2,Nu) - CG velocities in globals
%%%%%%%%%%%%%%%%%%%%%%%%%%%%%%%%%%%%%%%%%%%%%%%%%%%%%%%%%%%%%%%%%%%%%%%%%%
Vaa=Va; % axle velocities in locals
Vgg=Vg; % CG velocities in locals

% actual dimensions
Nu=size(PARSu,1);
Na=size(PARSa,1);

LL=PARSu(:,3);
XG=PARSu(:,4);
XX=LL-XG;

uu=zeros(2,Nu); 
nn=zeros(2,Nu);
for i=1:Nu
    c=cos(q(i+2));s=sin(q(i+2));
    uu(:,i)=[c,s]';
    nn(:,i)=[-s,c]';
end


Vj(:,1)=[qd(1),qd(2)]';
for i=1:Nu
    Vj(:,i+1)=Vj(:,i)-qd(i+2)*LL(i)*nn(:,i);%negative sign since working backwards
    Vg(:,i)=Vj(:,i)-qd(i+2)*XX(i)*nn(:,i);
    Vgx=dot(Vg(:,i),uu(:,i));Vgy=dot(Vg(:,i),nn(:,i));
    Vgg(:,i)=[Vgx;Vgy];
end

%velocities at axles 
for i=1:Na
    xa=PARSa(i,1);
    k=PARSa(i,2);
    Va(:,i)=Vj(:,k+1)+qd(k+2)*xa*nn(:,k);
    Vax=dot(Va(:,i),uu(:,k));Vay=dot(Va(:,i),nn(:,k));
    Vaa(:,i)=[Vax;Vay];
end

== matlab function manual_steer/double sat_tyre general model/double-general-lineartyre-variable/D ==
  data: D output
function D = calculate_D()

d1 = 10000;
d2 = 10000;

delta_kj = eye(3);
dj = [0, d1, d2, 0]';
D = zeros(5);

for k = 1:5
    for l = 1:5
        if k > 2 && l > 2
            if  l == k
                D(k, l) = (1 - delta_kj(1, k-2))*dj(k - 2) + (1 - delta_kj(3, k-2))*dj(k - 1);
            elseif l == k-1
                D(k, l) = -(1 - delta_kj(1, k-2))*dj(k - 2);
            elseif l == k+1
                D(k, l) = -(1 - delta_kj(3, k-2))*dj(k - 1);
            else
                D(k, l) = 0;
            end
        end
    end
end

end

== matlab function manual_steer/double sat_tyre general model/double-general-lineartyre-variable/M ==
  data: M output; q input
function M = calculate_M(q)

psi1 = q(3);
psi2 = q(4);
psi3 = q(5);

m1 = 11142;
m3 = 11142;
m2 = 7651; 
l_j1j2 = 11.4;
l_j2j3 = 9.4;
l_j1g1 = 5.862; 
l_j2g2 = 4.643; 
l_j3g3 = 5.538; 
iz1 = 143570; 
iz3 = 143570; 
iz2 = 37800;

l_kj = [l_j1g1, l_j1j2, l_j1j2;
             0, l_j2g2, l_j2j3;
             0,      0, l_j3g3;];
delta_kj = eye(3);
Jc = zeros(3, 5, 3);
for j = 1:3
    Jc(:, :, j) = [1, 0,  l_kj(1, j) * sin(psi1),  l_kj(2, j) * sin(psi2),  l_kj(3, j) * sin(psi3);
          0, 1, -l_kj(1, j) * cos(psi1), -l_kj(2, j) * cos(psi2), -l_kj(3, j) * cos(psi3);
          0, 0,          delta_kj(1, j),          delta_kj(2, j),          delta_kj(3, j);];
end

mj = [m1, m2, m3]';
izj = [iz1, iz2, iz3]';
Mj = zeros(3, 3, 3);
for j = 1:3
    Mj(:, :, j) = diag([mj(j), mj(j), izj(j)]);
end

M = zeros(5, 5);
for j = 1:3
    M = M + Jc(:, :, j)' * Mj(:, :, j) * Jc(:, :, j);
end

end

== matlab function manual_steer/single sat_tyre general model/ Motion Controller/discrete-time subsystem single/getU ==
  settings: updateMethod=DISCRETE
  data: U output; q input; qd input
function U = vx_conversion(q, qd)

% convert q and qd to vx6 needed for the driver model

% nominal point P of driver
xxp = 2;  
u1 = [cos(q(3)); sin(q(3))];
n1 = [-sin(q(3)); cos(q(3))];

% global velocity at front joint
vj1 = qd(1:2); 

% move to driver point
vp = vj1 - qd(3)*xxp*n1; 

% components in body axes (unit 1)
U = dot(vp, u1);

end
